simulink model "MicrostrainIMUTest01"  (Simulink 8.1)
settings: Solver=FixedStepDiscrete  StartTime=0.0  StopTime=inf  FixedStep=0.001  RelTol=1e-3
InitFcn:
  | IMU_Alignment_Params = [0 90 180];
libraries: xpcethercatlib x25
settings Model: Creator=bgbuss  LastModifiedBy=bgbuss  BufferReuse=off
settings DataIOCC: LimitDataPoints=off
settings OptimizationCC: BlockReduction=off  OptimizeBlockIOStorage=off  BufferReuse=off  ExpressionFolding=off  LocalBlockOutputs=off
settings DebuggingCC: FcnCallInpInsideContextMsg=EnableAllAsWarning
settings HardwareCC: ProdIntDivRoundTo=Zero  ProdEndianess=LittleEndian  ProdHWDeviceType=Generic->32-bit x86 compatible
settings RTWCC: SystemTargetFile=xpctarget.tlc  TemplateMakefile=xpc_default_tmf  Description=xPC Target  ProcessScript=xpctarget_make_rtw_hook  RTWCompilerOptimization=On
settings xpcTargetCC: TargetFcnLib=ansi_tfl_table_tmw.mat  CodeReplacementLibrary=XPC_BLAS  ParMdlRefBuildCompliant=on  ConcurrentExecutionCompliant=on  CombineSignalStateStructs=off  MATLABClassNameForMDSCustomization=xpcAperiodicCustomization  GRTInterface=on  GenerateAllocFcn=off  RL32LogBufSizeModifier=10000000  xPCTaskExecutionProfile=off  xPCRL32EventNumber=5000  xPCisModelTimeout=off  xPCModelTimeoutSecs=10  xPCLoadParamSetFile=off  xPCConcurrentTasks=off  xPCEnableSFAnimation=off

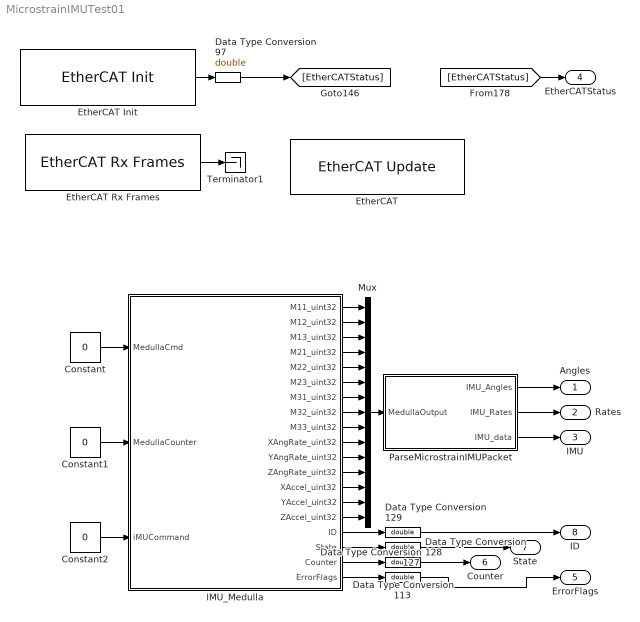
== system MicrostrainIMUTest01 ==
  Constant : Constant  Value=0
  Constant1 : Constant  Value=0
  Constant2 : Constant  Value=0
  Data Type Conversion{97,113,127..129} (5 alike) : DataTypeConversion  OutDataTypeStr=double
  EtherCAT : xpcethercatlib/EtherCAT Update   Priority=4  device_id=0  task_id_list=[1]  task_rates=[1]  task_priorities=[1500]
  EtherCAT Init : xpcethercatlib/EtherCAT Init   Priority=0  config_file='microstrain_imu_eni.xml'  device_id=0  pci_bus=4  pci_slot=4  enaDC=on  errRptLevel=0  sample_time=-1
  EtherCAT Rx Frames : xpcethercatlib/EtherCAT Rx Frames   Priority=1  device_id=0  sample_time=0
  IMU_Medulla : Subsystem
  Mux : Mux  Inputs=15
  ParseMicrostrainIMUPacket : Subsystem
  Terminator1 : Terminator
  Angles : Outport
  Rates : Outport  Port=2
  IMU : Outport  Port=3
  EtherCATStatus : Outport  Port=4
  ErrorFlags : Outport  Port=5
  Counter : Outport  Port=6
  State : Outport  Port=7
  ID : Outport  Port=8
  wires:
  ParseMicrostrainIMUPacket/1(IMU_Angles) -> Angles/1
  ParseMicrostrainIMUPacket/2(IMU_Rates) -> Rates/1
  ParseMicrostrainIMUPacket/3(IMU_data) -> IMU/1
  Mux/1 -> ParseMicrostrainIMUPacket/1(MedullaOutput)
  IMU_Medulla/1(M11_uint32) -> Mux/1
  IMU_Medulla/2(M12_uint32) -> Mux/2
  IMU_Medulla/3(M13_uint32) -> Mux/3
  IMU_Medulla/4(M21_uint32) -> Mux/4
  IMU_Medulla/5(M22_uint32) -> Mux/5
  IMU_Medulla/6(M23_uint32) -> Mux/6
  IMU_Medulla/7(M31_uint32) -> Mux/7
  IMU_Medulla/8(M32_uint32) -> Mux/8
  IMU_Medulla/9(M33_uint32) -> Mux/9
  IMU_Medulla/10(XAngRate_uint32) -> Mux/10
  IMU_Medulla/11(YAngRate_uint32) -> Mux/11
  IMU_Medulla/12(ZAngRate_uint32) -> Mux/12
  IMU_Medulla/13(XAccel_uint32) -> Mux/13
  IMU_Medulla/14(YAccel_uint32) -> Mux/14
  IMU_Medulla/15(ZAccel_uint32) -> Mux/15
  IMU_Medulla/19(ErrorFlags) -> Data Type Conversion127/1
  IMU_Medulla/18(Counter) -> Data Type Conversion113/1
  IMU_Medulla/17(State) -> Data Type Conversion128/1
  IMU_Medulla/16(ID) -> Data Type Conversion129/1
  Data Type Conversion129/1 -> ID/1
  Data Type Conversion128/1 -> State/1
  Data Type Conversion113/1 -> Counter/1
  Data Type Conversion127/1 -> ErrorFlags/1
  Constant/1 -> IMU_Medulla/1(MedullaCmd)
  Constant1/1 -> IMU_Medulla/2(MedullaCounter)
  Constant2/1 -> IMU_Medulla/3(iMUCommand)
  EtherCAT Rx Frames/1 -> Terminator1/1
  EtherCAT Init/1 -> Data Type Conversion97/1
  Data Type Conversion97/1 -> [EtherCATStatus]
  [EtherCATStatus] -> EtherCATStatus/1

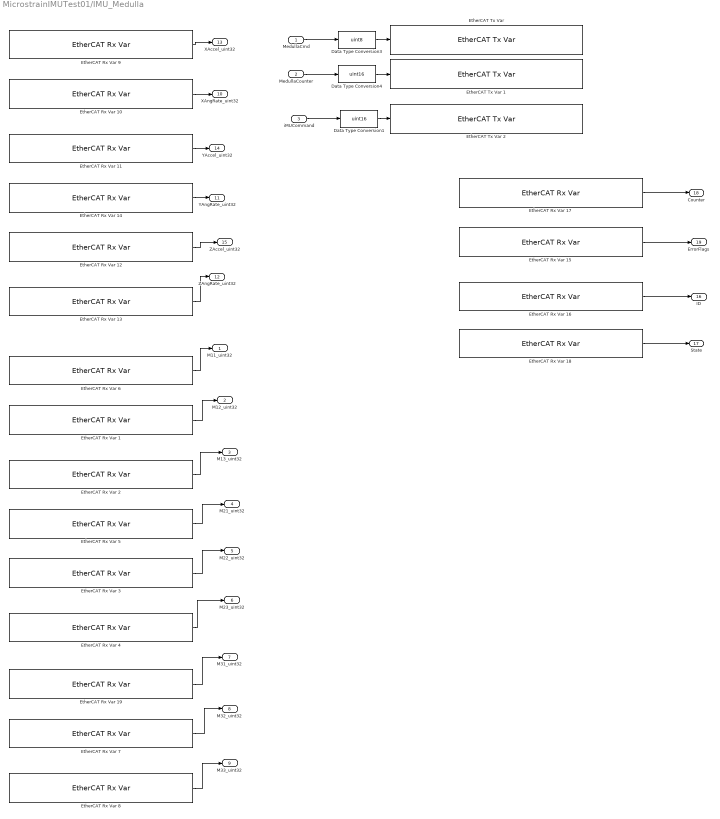
== system MicrostrainIMUTest01/IMU_Medulla ==
  MedullaCmd : Inport
  MedullaCounter : Inport  Port=2
  iMUCommand : Inport  Port=3
  Data Type Conversion1 : DataTypeConversion  OutDataTypeStr=uint16
  Data Type Conversion3 : DataTypeConversion  OutDataTypeStr=uint8
  Data Type Conversion4 : DataTypeConversion  OutDataTypeStr=uint16
  EtherCAT Rx Var 1 : xpcethercatlib/EtherCAT Rx Var   Priority=2  sig_name=Box 2 (ATRIAS 2.1 Microstrain IMU (Medulla 1.5)).M.M12  sig_offset=720  sig_type=uint32  type_size=32  sig_dim=1  device_id=0  sample_time=0.001000
  EtherCAT Rx Var 10 : xpcethercatlib/EtherCAT Rx Var   Priority=2  sig_name=Box 2 (ATRIAS 2.1 Microstrain IMU (Medulla 1.5)).Xaxes.XAngRate  sig_offset=496  sig_type=uint32  type_size=32  sig_dim=1  device_id=0  sample_time=0.001000
  EtherCAT Rx Var 11 : xpcethercatlib/EtherCAT Rx Var   Priority=2  sig_name=Box 2 (ATRIAS 2.1 Microstrain IMU (Medulla 1.5)).Yaxes.YAccel  sig_offset=592  sig_type=uint32  type_size=32  sig_dim=1  device_id=0  sample_time=0.001000
  EtherCAT Rx Var 12 : xpcethercatlib/EtherCAT Rx Var   Priority=2  sig_name=Box 2 (ATRIAS 2.1 Microstrain IMU (Medulla 1.5)).Zaxes.ZAccel  sig_offset=656  sig_type=uint32  type_size=32  sig_dim=1  device_id=0  sample_time=0.001000
  EtherCAT Rx Var 13 : xpcethercatlib/EtherCAT Rx Var   Priority=2  sig_name=Box 2 (ATRIAS 2.1 Microstrain IMU (Medulla 1.5)).Zaxes.ZAngRate  sig_offset=624  sig_type=uint32  type_size=32  sig_dim=1  device_id=0  sample_time=0.001000
  EtherCAT Rx Var 14 : xpcethercatlib/EtherCAT Rx Var   Priority=2  sig_name=Box 2 (ATRIAS 2.1 Microstrain IMU (Medulla 1.5)).Yaxes.YAngRate  sig_offset=560  sig_type=uint32  type_size=32  sig_dim=1  device_id=0  sample_time=0.001000
  EtherCAT Rx Var 15 : xpcethercatlib/EtherCAT Rx Var   Priority=2  sig_name=Box 2 (ATRIAS 2.1 Microstrain IMU (Medulla 1.5)).uController Status.Error Flags  sig_offset=488  sig_type=uint8  type_size=8  sig_dim=1  device_id=0  sample_time=0.001000
  EtherCAT Rx Var 16 : xpcethercatlib/EtherCAT Rx Var   Priority=2  sig_name=Box 2 (ATRIAS 2.1 Microstrain IMU (Medulla 1.5)).uController Status.ID  sig_offset=464  sig_type=uint8  type_size=8  sig_dim=1  device_id=0  sample_time=0.001000
  EtherCAT Rx Var 17 : xpcethercatlib/EtherCAT Rx Var   Priority=2  sig_name=Box 2 (ATRIAS 2.1 Microstrain IMU (Medulla 1.5)).uController Status.Counter  sig_offset=480  sig_type=uint8  type_size=8  sig_dim=1  device_id=0  sample_time=0.001000
  EtherCAT Rx Var 18 : xpcethercatlib/EtherCAT Rx Var   Priority=2  sig_name=Box 2 (ATRIAS 2.1 Microstrain IMU (Medulla 1.5)).uController Status.State  sig_offset=472  sig_type=uint8  type_size=8  sig_dim=1  device_id=0  sample_time=0.001000
  EtherCAT Rx Var 19 : xpcethercatlib/EtherCAT Rx Var   Priority=2  sig_name=Box 2 (ATRIAS 2.1 Microstrain IMU (Medulla 1.5)).M.M31  sig_offset=880  sig_type=uint32  type_size=32  sig_dim=1  device_id=0  sample_time=0.001000
  EtherCAT Rx Var 2 : xpcethercatlib/EtherCAT Rx Var   Priority=2  sig_name=Box 2 (ATRIAS 2.1 Microstrain IMU (Medulla 1.5)).M.M13  sig_offset=752  sig_type=uint32  type_size=32  sig_dim=1  device_id=0  sample_time=0.001000
  EtherCAT Rx Var 3 : xpcethercatlib/EtherCAT Rx Var   Priority=2  sig_name=Box 2 (ATRIAS 2.1 Microstrain IMU (Medulla 1.5)).M.M22  sig_offset=816  sig_type=uint32  type_size=32  sig_dim=1  device_id=0  sample_time=0.001000
  EtherCAT Rx Var 4 : xpcethercatlib/EtherCAT Rx Var   Priority=2  sig_name=Box 2 (ATRIAS 2.1 Microstrain IMU (Medulla 1.5)).M.M23  sig_offset=848  sig_type=uint32  type_size=32  sig_dim=1  device_id=0  sample_time=0.001000
  EtherCAT Rx Var 5 : xpcethercatlib/EtherCAT Rx Var   Priority=2  sig_name=Box 2 (ATRIAS 2.1 Microstrain IMU (Medulla 1.5)).M.M21  sig_offset=784  sig_type=uint32  type_size=32  sig_dim=1  device_id=0  sample_time=0.001000
  EtherCAT Rx Var 6 : xpcethercatlib/EtherCAT Rx Var   Priority=2  sig_name=Box 2 (ATRIAS 2.1 Microstrain IMU (Medulla 1.5)).M.M11  sig_offset=688  sig_type=uint32  type_size=32  sig_dim=1  device_id=0  sample_time=0.001000
  EtherCAT Rx Var 7 : xpcethercatlib/EtherCAT Rx Var   Priority=2  sig_name=Box 2 (ATRIAS 2.1 Microstrain IMU (Medulla 1.5)).M.M32  sig_offset=912  sig_type=uint32  type_size=32  sig_dim=1  device_id=0  sample_time=0.001000
  EtherCAT Rx Var 8 : xpcethercatlib/EtherCAT Rx Var   Priority=2  sig_name=Box 2 (ATRIAS 2.1 Microstrain IMU (Medulla 1.5)).M.M33  sig_offset=944  sig_type=uint32  type_size=32  sig_dim=1  device_id=0  sample_time=0.001000
  EtherCAT Rx Var 9 : xpcethercatlib/EtherCAT Rx Var   Priority=2  sig_name=Box 2 (ATRIAS 2.1 Microstrain IMU (Medulla 1.5)).Xaxes.XAccel  sig_offset=528  sig_type=uint32  type_size=32  sig_dim=1  device_id=0  sample_time=0.001000
  "EtherCAT Tx Var " : xpcethercatlib/EtherCAT Tx Var   Priority=3  sig_name=Box 2 (ATRIAS 2.1 Microstrain IMU (Medulla 1.5)).uControllerInput.Command  sig_offset=464  sig_type=uint8  type_size=8  sig_dim=1  device_id=0  sample_time=0.001000
  EtherCAT Tx Var 1 : xpcethercatlib/EtherCAT Tx Var   Priority=3  sig_name=Box 2 (ATRIAS 2.1 Microstrain IMU (Medulla 1.5)).uControllerInput.Counter  sig_offset=472  sig_type=uint16  type_size=16  sig_dim=1  device_id=0  sample_time=0.001000
  EtherCAT Tx Var 2 : xpcethercatlib/EtherCAT Tx Var   Priority=3  sig_name=Box 2 (ATRIAS 2.1 Microstrain IMU (Medulla 1.5)).uControllerInput.IMU_cmd  sig_offset=488  sig_type=uint16  type_size=16  sig_dim=1  device_id=0  sample_time=0.001000
  M11_uint32 : Outport
  M12_uint32 : Outport  Port=2
  M13_uint32 : Outport  Port=3
  M21_uint32 : Outport  Port=4
  M22_uint32 : Outport  Port=5
  M23_uint32 : Outport  Port=6
  M31_uint32 : Outport  Port=7
  M32_uint32 : Outport  Port=8
  M33_uint32 : Outport  Port=9
  XAngRate_uint32 : Outport  Port=10
  YAngRate_uint32 : Outport  Port=11
  ZAngRate_uint32 : Outport  Port=12
  XAccel_uint32 : Outport  Port=13
  YAccel_uint32 : Outport  Port=14
  ZAccel_uint32 : Outport  Port=15
  ID : Outport  Port=16
  State : Outport  Port=17
  Counter : Outport  Port=18
  ErrorFlags : Outport  Port=19
  wires:
  EtherCAT Rx Var 18/1 -> State/1
  EtherCAT Rx Var 16/1 -> ID/1
  EtherCAT Rx Var 15/1 -> ErrorFlags/1
  EtherCAT Rx Var 17/1 -> Counter/1
  Data Type Conversion1/1 -> EtherCAT Tx Var 2/1
  iMUCommand/1 -> Data Type Conversion1/1
  MedullaCounter/1 -> Data Type Conversion4/1
  MedullaCmd/1 -> Data Type Conversion3/1
  Data Type Conversion4/1 -> EtherCAT Tx Var 1/1
  Data Type Conversion3/1 -> "EtherCAT Tx Var "/1
  EtherCAT Rx Var 8/1 -> M33_uint32/1
  EtherCAT Rx Var 7/1 -> M32_uint32/1
  EtherCAT Rx Var 19/1 -> M31_uint32/1
  EtherCAT Rx Var 4/1 -> M23_uint32/1
  EtherCAT Rx Var 3/1 -> M22_uint32/1
  EtherCAT Rx Var 5/1 -> M21_uint32/1
  EtherCAT Rx Var 2/1 -> M13_uint32/1
  EtherCAT Rx Var 1/1 -> M12_uint32/1
  EtherCAT Rx Var 6/1 -> M11_uint32/1
  EtherCAT Rx Var 13/1 -> ZAngRate_uint32/1
  EtherCAT Rx Var 12/1 -> ZAccel_uint32/1
  EtherCAT Rx Var 14/1 -> YAngRate_uint32/1
  EtherCAT Rx Var 11/1 -> YAccel_uint32/1
  EtherCAT Rx Var 10/1 -> XAngRate_uint32/1
  EtherCAT Rx Var 9/1 -> XAccel_uint32/1

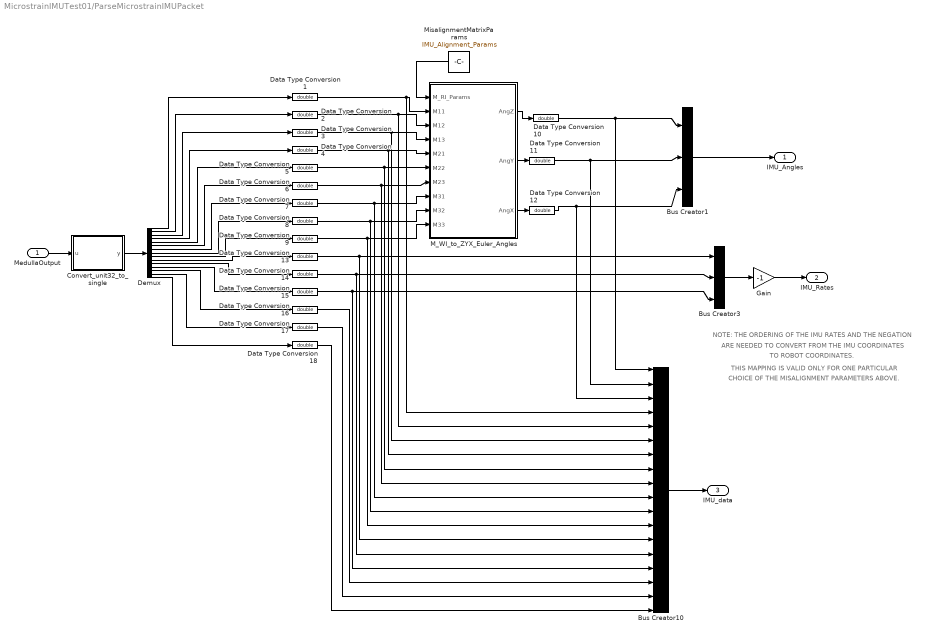
== system MicrostrainIMUTest01/ParseMicrostrainIMUPacket ==
  note: CHOICE OF THE MISALIGNMENT PARAMETERS ABOVE.
  note: THIS MAPPING IS VALID ONLY FOR ONE PARTICULAR
  note: TO ROBOT COORDINATES.
  note: ARE NEEDED TO CONVERT FROM THE IMU COORDINATES
  note: NOTE: THE ORDERING OF THE IMU RATES AND THE NEGATION
  MedullaOutput : Inport
  Bus Creator1 : BusCreator  Inputs=3
  Bus Creator10 : BusCreator  Inputs=18
  Bus Creator3 : BusCreator  Inputs=3
  Convert_unit32_to_single : MATLAB Function  TreatAsAtomicUnit=on
  Data Type Conversion{1..18} (18 alike) : DataTypeConversion  OutDataTypeStr=double
  Demux : Demux  Outputs=15
  Gain : Gain  Gain=-1
  M_WI_to_ZYX_Euler_Angles : MATLAB Function  TreatAsAtomicUnit=on
  MisalignmentMatrixParams : Constant  Value=IMU_Alignment_Params
  IMU_Angles : Outport
  IMU_Rates : Outport  Port=2
  IMU_data : Outport  Port=3
  wires:
  Gain/1 -> IMU_Rates/1
  Bus Creator3/1 -> Gain/1
  Convert_unit32_to_single/1(y) -> Demux/1
  MedullaOutput/1 -> Convert_unit32_to_single/1(u)
  M_WI_to_ZYX_Euler_Angles/1(AngZ) -> Data Type Conversion10/1
  M_WI_to_ZYX_Euler_Angles/2(AngY) -> Data Type Conversion11/1
  M_WI_to_ZYX_Euler_Angles/3(AngX) -> Data Type Conversion12/1
  Data Type Conversion1/1 -> M_WI_to_ZYX_Euler_Angles/2(M11), Bus Creator10/4
  Data Type Conversion2/1 -> M_WI_to_ZYX_Euler_Angles/3(M12), Bus Creator10/5
  Data Type Conversion3/1 -> M_WI_to_ZYX_Euler_Angles/4(M13), Bus Creator10/6
  Data Type Conversion4/1 -> M_WI_to_ZYX_Euler_Angles/5(M21), Bus Creator10/7
  Data Type Conversion5/1 -> M_WI_to_ZYX_Euler_Angles/6(M22), Bus Creator10/8
  Data Type Conversion6/1 -> M_WI_to_ZYX_Euler_Angles/7(M23), Bus Creator10/9
  Data Type Conversion7/1 -> M_WI_to_ZYX_Euler_Angles/8(M31), Bus Creator10/10
  Data Type Conversion8/1 -> M_WI_to_ZYX_Euler_Angles/9(M32), Bus Creator10/11
  Data Type Conversion9/1 -> M_WI_to_ZYX_Euler_Angles/10(M33), Bus Creator10/12
  Data Type Conversion10/1 -> Bus Creator10/1, Bus Creator1/1
  Data Type Conversion11/1 -> Bus Creator10/2, Bus Creator1/2
  Data Type Conversion12/1 -> Bus Creator10/3, Bus Creator1/3
  Data Type Conversion13/1 -> Bus Creator10/13, Bus Creator3/1
  Data Type Conversion14/1 -> Bus Creator3/2, Bus Creator10/14
  Data Type Conversion15/1 -> Bus Creator3/3, Bus Creator10/15
  MisalignmentMatrixParams/1 -> M_WI_to_ZYX_Euler_Angles/1(M_RI_Params)
  Demux/1 -> Data Type Conversion1/1
  Demux/2 -> Data Type Conversion2/1
  Demux/3 -> Data Type Conversion3/1
  Demux/4 -> Data Type Conversion4/1
  Demux/5 -> Data Type Conversion5/1
  Demux/6 -> Data Type Conversion6/1
  Demux/7 -> Data Type Conversion7/1
  Demux/8 -> Data Type Conversion8/1
  Demux/9 -> Data Type Conversion9/1
  Demux/10 -> Data Type Conversion13/1
  Demux/11 -> Data Type Conversion14/1
  Demux/12 -> Data Type Conversion15/1
  Demux/13 -> Data Type Conversion16/1
  Demux/14 -> Data Type Conversion17/1
  Demux/15 -> Data Type Conversion18/1
  Data Type Conversion18/1 -> Bus Creator10/18
  Data Type Conversion17/1 -> Bus Creator10/17
  Data Type Conversion16/1 -> Bus Creator10/16
  Bus Creator1/1 -> IMU_Angles/1
  Bus Creator10/1 -> IMU_data/1

== matlab function ParseMicrostrainIMUPacket/Convert_unit32_to_single ==
  data: u input uint32; y output single
function y = fcn(u)
%#codegen
y = typecast(u, 'single');

== matlab function ParseMicrostrainIMUPacket/M_WI_to_ZYX_Euler_Angles ==
  data: M_RI_Params input double; AngZ output double; M11 input double; M12 input double; M13 input double; M21 input double; M22 input double; M23 input double; M31 input double; M32 input double; M33 input double; AngY output double; AngX output double
function [AngZ,AngY,AngX] = fcn(M_RI_Params,M11,M12,M13,M21,M22,M23,M31,M32,M33)
%#codegen
AngZ = 0;
AngY = 0;
AngX = 0;
%Inputs are the three Euler angles (ZYX convention) in degrees which parametrize the
%matrix M_RI, and the 9 elements of the M_WI matrix reported by the IMU
M_RI_Z_rad = M_RI_Params(1)*pi/180;
M_RI_Y_rad = M_RI_Params(2)*pi/180;
M_RI_X_rad = M_RI_Params(3)*pi/180;

%Form the M_WI matrix from the inputs
M_WI = [M11,M12,M13;M21,M22,M23;M31,M32,M33];  
M_IW = M_WI.';
%Form the M_RI matrix from the paramters
M_RI = RotZ(M_RI_Z_rad)*RotY(M_RI_Y_rad)*RotX(M_RI_X_rad);
%Create the matrix that takes us from world frame 1 (z-down) to world frame
%2 (z-up)
M_W_W2 = [0 1 0;1 0 0;0 0 -1]; 

M_RW = M_IW*M_RI; %Relationship between robot frame and world frame 1 (z-down)

M_RW2 = M_W_W2*M_RW; %Relationship between robot frame and world frame 2 (z-up)

[AngX,AngY,AngZ] = M_to_ZYX(M_RW2);

end

function [AngX_out,AngY_out,AngZ_out] = M_to_ZYX(M_RW_in)
% M_to_ZYX.m
% Author: Kevin Galloway
% Date: 29AUG12
%
% Summary: This function takes a matrix (or array of matrices) M_RW_in and
% returns the Euler angles based on the ZYX convention. AngX refers to
% rotation around the X axis, AngY refers to rotation about the Y axis, and
% AngZ refers to rotation about the Z axis. If M_RW_in is an array of
% matrices (i.e. a multidimensional array), then AngX, AngY and AngZ
% will be vectors.
M31_RW_in = M_RW_in(3,1);
M32_RW_in = M_RW_in(3,2);
M33_RW_in = M_RW_in(3,3);
M21_RW_in = M_RW_in(2,1);
M11_RW_in = M_RW_in(1,1);
AngY_out = asin(-M31_RW_in);
AngX_out = atan2(M32_RW_in,M33_RW_in);
AngZ_out = atan2(M21_RW_in,M11_RW_in);
end

function M_X = RotX(phi)
M_X = [1 0 0; 0 cos(phi) -sin(phi); 0 sin(phi) cos(phi)];
end

function M_Y = RotY(theta)
M_Y = [cos(theta) 0 sin(theta); 0 1 0; -sin(theta) 0 cos(theta)];
end

function M_Z = RotZ(psi)
M_Z = [cos(psi) -sin(psi) 0; sin(psi) cos(psi) 0; 0 0 1];
end
